simulink model "Stateflow_Model_for_if_test"  (R2013b)
settings: Solver=ode4  StartTime=0.0  StopTime=10.0  FixedStep=dT  RelTol=1e-3
values from neighbouring files (symbols this model uses):
  a_in = 2    [Stateflow_Model_execute.m]
  b = 2    [Stateflow_Model_execute.m]
  c = 3    [Stateflow_Model_execute.m]
settings Model: Creator=daltdoer  LastModifiedBy=daltdoer

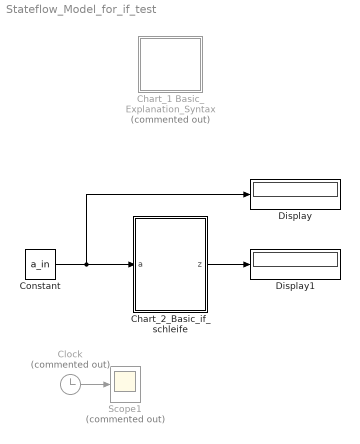
== system Stateflow_Model_for_if_test ==
  Chart_1 Basic_Explanation_Syntax : Stateflow chart  Commented=on  TreatAsAtomicUnit=on
  Chart_2_Basic_if_schleife : Stateflow chart  TreatAsAtomicUnit=on
  Clock : Clock  Commented=on
  Constant : Constant  Value=a_in
  Display : Display
  Display1 : Display
  Scope1 : Scope  Commented=on
  wires:
  Constant/1 -> Chart_2_Basic_if_schleife/1(a), Display/1
  Chart_2_Basic_if_schleife/1(z) -> Display1/1
  Clock/1 -> Scope1/1

== stateflow chart Stateflow_Model_for_if_test/Chart_1 Basic_Explanation_Syntax ==
  note: Default Transition:
      | legt fest, welcher Zustand nach erstmaliger Ausführung aktiv sein soll
  state Name Zustand/
    entry: Aktion 1; %wenn der Zustand aktiviert wird
    during: Aktion 2; %wenn der Zustand aktiv ist (und das Chart ausgeführt wird)
    exit: Aktion 3; %wenn der Zustand verlassen wird
    on event Aktion 4; %wenn der Zustand aktiv ist und das angegebene Ereignis auftritt
  state Name Zustand 2/
    entry: Aktion 1; %wenn der Zustand aktiviert wird
    during: Aktion 2; %wenn der Zustand aktiv ist (und das Chart ausgeführt wird)
    exit: Aktion 3; %wenn der Zustand verlassen wird
    on event Aktion 4; %wenn der Zustand aktiv ist und das angegebene Ereignis auftritt
  note: Ein Transitionslabel besitzt die Syntax:
  note: Transition ist gültig, WENN:
      | -Ausgangszustand aktiv, insofern kein Ereignis oder Bedingung angegeben
      | -das Ereignis "event" eintritt
      | -die angegebene Bedingung "condition" TRUE ist
  (default) -> Name Zustand : u
  Name Zustand -> Name Zustand 2 : event[condition==1]{conditionAction}/transitionAction

== stateflow chart Stateflow_Model_for_if_test/Chart_2_Basic_if_schleife ==
  note: Flussdiagramm mit if Abfrage
  note: Ein Transitionslabel besitzt die Syntax:
      |
      | event[condition==1]{conditionAction}/transitionAction
  note: Transition ist gültig, WENN:
      | -Ausgangszustand aktiv, insofern kein Ereignis oder Bedingung angegeben
      | -das Ereignis "event" eintritt
      | -die angegebene Bedingung "condition" TRUE ist
  (default) -> (junction 12)
  (junction 12) -> (junction 14) [order 1] : [a>b]{z=1}
  (junction 14) -> (junction 18) [order 1] : [a>c]{z=3}
  (junction 14) -> (junction 18) [order 2] : {z=4}
  (junction 12) -> (junction 18) [order 2] : {z=5}
  data: a input double; b parameter double; c parameter double; z output double
